simulink library "kukaslxctrl"  (R2016b)
settings: Solver=ode45  StartTime=0.0  StopTime=10.0  RelTol=1e-3  EnableMultiTasking=on
undefined symbols (not defined in the file): dcpctrl, getInitState, Standard_Devices, UDP_Protocol
libraries: simulink x2, sldrtlib x2
settings Model: Creator=julianleland  LastModifiedBy=dcp
settings DataIOCC: LimitDataPoints=on
settings OptimizationCC: LifeSpan=inf
settings DebuggingCC: AllowSymbolicDim=off  SFUnexpectedBacktrackingDiag=warning  SFNoUnconditionalDefaultTransitionDiag=warning  SFExecutionAtInitializationDiag=none
settings GRTTargetCC: TargetLangStandard=C89/C90 (ANSI)  GeneratePreprocessorConditionals=Disable all
settings ConfigComp: CovMetricSettings=dw  CovHtmlReporting=on  CovSaveCumulativeToWorkspaceVar=on  CovSaveSingleToWorkspaceVar=on  CovExternalEMLEnable=off

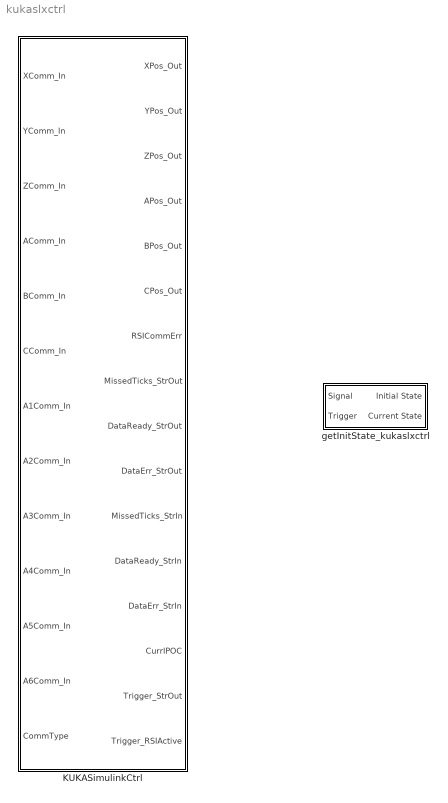
== system kukaslxctrl ==
  KUKASimulinkCtrl : Subsystem  mask(KUKASimulinkCtrl){}
      mask help:
      | This block produces an interface for communicating with KUKA robots using KRC4 and RSI. This block is currently in development, so not all inputs and outputs are usable yet!
      |
      | Notes:
      |  - This system assumes relative motion commands by default: e.g., a command of 1 sent to XComm_In will tell the KUKA to move at 1 mm/.004 sec (= 250 mm/sec - don't do this, too fast!!).
      |  - You will need to configure the Stream Input and Stream Output blocks inside this block - as well as the KUKA RSI files - to match your network configuration.
      |  - This block requires the Simulink Desktop Real-Time blockset to operate.
      |
      | Please see help for detailed information on inputs and outputs.
      mask Help:
      | INPUTS:
      |  - XComm_In, etc.: Task-space (XYZABC) commands to send to KUKA.
      |  - A1Comm_In, etc.: Joint-space commands to send to KUKA. NOT CURRENTLY FUNCTIONAL.
      |  - CommType: Flag to indicate whether using task-space or joint-space commands. NOT CURRENTLY FUNCTIONAL.
      | 
      | OUTPUTS:
      |  - XPos_Out, etc.: Task-space positions.
      |  - RSICommErr: Eventually will report if there's an error in creating an RSI packet - currently does nothing.
      |  - MissedTicks_StrOut: Missed ticks from UDP Stream Output block.
      |  - DataReady_StrOut: Data Ready flag from UDP Stream Output block.
      |  - DataErr_StrOut: Data Error flag from UDP Stream Output block.
      |  - MissedTicks_StrIn: Missed ticks from UDP Stream Input block.
      |  - DataReady_StrIn: Data Ready flag from UDP Stream Input block.
      |  - DataErr_StrIn: Data Error flag from UDP Stream Input block.
      |  - CurrIPOC: Reports the IPOC from the last received packet.
      |  - Trigger_StrOut: Trigger flag indicating when stream output has been turned on (after system has received first packet from KUKA).
      |  - Trigger_RSIActive: Trigger flag indicating when a numerical (non-NaN) IPOC value has been received.
      | 
      | DEPENDENCIES: Requires Simulink Desktop Real-Time.
      | 
      | NOTES: None.
  getInitState_kukaslxctrl : Subsystem  AncestorBlock=dcpctrl/getInitState  mask(Initial State Capture){}
      mask help:
      | Captures state of signal at time that trigger input is set high. Outputs captured state, as well as current signal. A common use of this block is to capture the initial state of a signal, and then subtract the initial state from the current state, giving a measure of how much a signal has changed over time.
      |
      | INPUTS:
      |  - Signal: Signal to capture state of.
      |  - Trigger: Signal carrying trigger to set state capture. Captures on rising edge. A step signal is a good choice for a trigger.
      |
      | OUTPUTS:
      |  - Initial State: State of signal at time when trigger rising edge is detected.
      |  - Current State: Signal (passed through).
      |
      | DEPENDENCIES: None
      |
      | NOTES: This is a convenience function included to support the example kukaslxctrl.slx

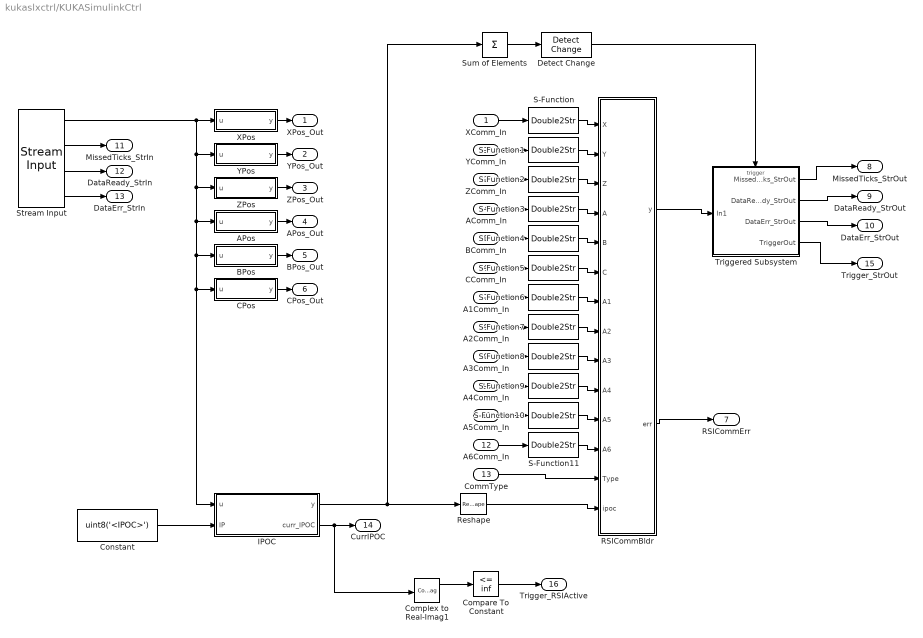
== system kukaslxctrl/KUKASimulinkCtrl ==
  XComm_In : Inport
  YComm_In : Inport  Port=2
  ZComm_In : Inport  Port=3
  AComm_In : Inport  Port=4
  BComm_In : Inport  Port=5
  CComm_In : Inport  Port=6
  A1Comm_In : Inport  Port=7
  A2Comm_In : Inport  Port=8
  A3Comm_In : Inport  Port=9
  A4Comm_In : Inport  Port=10
  A5Comm_In : Inport  Port=11
  A6Comm_In : Inport  Port=12
  CommType : Inport  Port=13
  APos : MATLAB Function  TreatAsAtomicUnit=on
  BPos : MATLAB Function  TreatAsAtomicUnit=on
  CPos : MATLAB Function  TreatAsAtomicUnit=on
  Compare To Constant : simulink/Logic and Bit Operations/Compare To Constant  relop=<=  const=inf  OutDataTypeStr=boolean
  Complex to Real-Imag1 : ComplexToRealImag
  Constant : Constant  Value=uint8('<IPOC>')
  Detect Change : simulink/Logic and Bit Operations/Detect Change  vinit=0  OutDataTypeStr=boolean
  IPOC : MATLAB Function  TreatAsAtomicUnit=on
  RSICommBldr : MATLAB Function  TreatAsAtomicUnit=on
  Reshape : Reshape
  S-Function{,1..11} (12 alike) : S-Function  FunctionName=Double2Str  SFunctionDeploymentMode=off  EnableBusSupport=off
  Stream Input : sldrtlib/Stream Input  SampleTime=-1  MaxMissedTicks=10  ShowMissedTicks=on  YieldWhenWaiting=on  DrvName=Standard_Devices/UDP_Protocol  DrvAddress=27277  DrvOptions=[174338149 53453]  DataTypes='238*uint16'  FormatString=repmat('%c',1,238)  Terminator='/Rob>'  ShowReady=on  ShowError=on
      settings: AttributesFormatString=Standard Devices\nUDP Protocol [6A8Dh]
  Sum of Elements : Sum  Inputs=+  CollapseMode=Specified dimension  CollapseDim=2
  Triggered Subsystem : Subsystem  TreatAsAtomicUnit=on
  XPos : MATLAB Function  TreatAsAtomicUnit=on
  YPos : MATLAB Function  TreatAsAtomicUnit=on
  ZPos : MATLAB Function  TreatAsAtomicUnit=on
  XPos_Out : Outport
  YPos_Out : Outport  Port=2
  ZPos_Out : Outport  Port=3
  APos_Out : Outport  Port=4
  BPos_Out : Outport  Port=5
  CPos_Out : Outport  Port=6
  RSICommErr : Outport  Port=7
  MissedTicks_StrOut : Outport  Port=8
  DataReady_StrOut : Outport  Port=9
  DataErr_StrOut : Outport  Port=10
  MissedTicks_StrIn : Outport  Port=11
  DataReady_StrIn : Outport  Port=12
  DataErr_StrIn : Outport  Port=13
  CurrIPOC : Outport  Port=14
  Trigger_StrOut : Outport  Port=15
  Trigger_RSIActive : Outport  Port=16
  wires:
  YComm_In/1 -> S-Function1/1
  BPos/1(y) -> BPos_Out/1
  CComm_In/1 -> S-Function5/1
  ZComm_In/1 -> S-Function2/1
  AComm_In/1 -> S-Function3/1
  BComm_In/1 -> S-Function4/1
  A6Comm_In/1 -> S-Function11/1
  RSICommBldr/2(err) -> RSICommErr/1
  A5Comm_In/1 -> S-Function10/1
  XPos/1(y) -> XPos_Out/1
  A2Comm_In/1 -> S-Function7/1
  A4Comm_In/1 -> S-Function9/1
  APos/1(y) -> APos_Out/1
  A3Comm_In/1 -> S-Function8/1
  YPos/1(y) -> YPos_Out/1
  A1Comm_In/1 -> S-Function6/1
  ZPos/1(y) -> ZPos_Out/1
  XComm_In/1 -> S-Function/1
  CPos/1(y) -> CPos_Out/1
  Stream Input/3 -> DataReady_StrIn/1
  S-Function/1 -> RSICommBldr/1(X)
  Stream Input/2 -> MissedTicks_StrIn/1
  Stream Input/1 -> IPOC/1(u), CPos/1(u), BPos/1(u), APos/1(u), ZPos/1(u), YPos/1(u), XPos/1(u)
  RSICommBldr/1(y) -> Triggered Subsystem/1(In1)
  IPOC/1(y) -> Sum of Elements/1, Reshape/1
  Constant/1 -> IPOC/2(IP)
  S-Function1/1 -> RSICommBldr/2(Y)
  S-Function2/1 -> RSICommBldr/3(Z)
  S-Function3/1 -> RSICommBldr/4(A)
  S-Function4/1 -> RSICommBldr/5(B)
  S-Function5/1 -> RSICommBldr/6(C)
  S-Function6/1 -> RSICommBldr/7(A1)
  S-Function7/1 -> RSICommBldr/8(A2)
  S-Function8/1 -> RSICommBldr/9(A3)
  S-Function9/1 -> RSICommBldr/10(A4)
  S-Function10/1 -> RSICommBldr/11(A5)
  S-Function11/1 -> RSICommBldr/12(A6)
  Triggered Subsystem/1(MissedTicks_StrOut) -> MissedTicks_StrOut/1
  Triggered Subsystem/2(DataReady_StrOut) -> DataReady_StrOut/1
  Triggered Subsystem/3(DataErr_StrOut) -> DataErr_StrOut/1
  Stream Input/4 -> DataErr_StrIn/1
  IPOC/2(curr_IPOC) -> Complex to Real-Imag1/1, CurrIPOC/1
  Reshape/1 -> RSICommBldr/14(ipoc)
  CommType/1 -> RSICommBldr/13(Type)
  Triggered Subsystem/4(TriggerOut) -> Trigger_StrOut/1
  Detect Change/1 -> Triggered Subsystem/Trigger
  Sum of Elements/1 -> Detect Change/1
  Compare To Constant/1 -> Trigger_RSIActive/1
  Complex to Real-Imag1/1 -> Compare To Constant/1

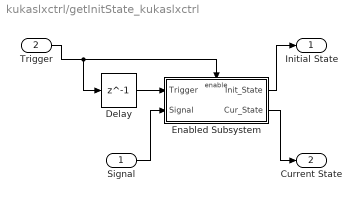
== system kukaslxctrl/getInitState_kukaslxctrl ==
  Signal : Inport
  Trigger : Inport  Port=2
  Delay : Delay  DelayLength=1  InitialCondition=0
  Enabled Subsystem : Subsystem  TreatAsAtomicUnit=on
  Initial State : Outport
  Current State : Outport  Port=2
  wires:
  Delay/1 -> Enabled Subsystem/1(Trigger)
  Trigger/1 -> Enabled Subsystem/Enable, Delay/1
  Enabled Subsystem/2(Cur_State) -> Current State/1
  Enabled Subsystem/1(Init_State) -> Initial State/1
  Signal/1 -> Enabled Subsystem/2(Signal)

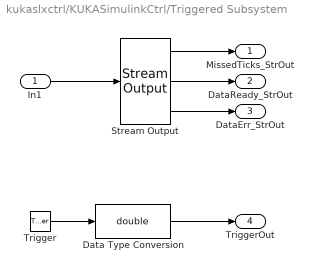
== system kukaslxctrl/KUKASimulinkCtrl/Triggered Subsystem ==
  In1 : Inport
  Trigger : TriggerPort  VariantControl=Variant  ShowOutputPort=on
  Data Type Conversion : DataTypeConversion  OutDataTypeStr=double
  Stream Output : sldrtlib/Stream Output  SampleTime=inf  MaxMissedTicks=10  ShowMissedTicks=on  YieldWhenWaiting=off  DrvName=Standard_Devices/UDP_Protocol  DrvAddress=27277  DrvOptions=[174338149 53453]  PortSizes=282  FormatString=repmat('%c',1,282)  ShowReady=on  ShowError=on  InitialValue=[]  FinalValue=[]
      settings: AttributesFormatString=Standard Devices\nUDP Protocol [6A8Dh]
  MissedTicks_StrOut : Outport
  DataReady_StrOut : Outport  Port=2
  DataErr_StrOut : Outport  Port=3
  TriggerOut : Outport  Port=4
  wires:
  Stream Output/1 -> MissedTicks_StrOut/1
  Stream Output/2 -> DataReady_StrOut/1
  Stream Output/3 -> DataErr_StrOut/1
  In1/1 -> Stream Output/1
  Data Type Conversion/1 -> TriggerOut/1
  Trigger/1 -> Data Type Conversion/1

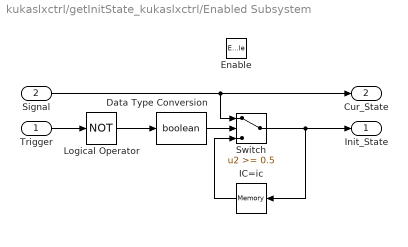
== system kukaslxctrl/getInitState_kukaslxctrl/Enabled Subsystem ==
  Trigger : Inport
  Signal : Inport  Port=2
  Enable : EnablePort  StatesWhenEnabling=reset
  Data Type Conversion : DataTypeConversion  OutDataTypeStr=boolean
  IC=ic : Memory  LinearizeAsDelay=on
  Logical Operator : Logic  Operator=NOT  AllPortsSameDT=off  OutDataTypeStr=boolean
  Switch : Switch  Threshold=0.5  SaturateOnIntegerOverflow=on  InputSameDT=on
  Init_State : Outport
  Cur_State : Outport  Port=2
  wires:
  Signal/1 -> Switch/1, Cur_State/1
  Logical Operator/1 -> Data Type Conversion/1
  IC=ic/1 -> Switch/3
  Switch/1 -> Init_State/1, IC=ic/1
  Data Type Conversion/1 -> Switch/2
  Trigger/1 -> Logical Operator/1

== matlab function kukaslxctrl/KUKASimulinkCtrl/XPos ==
  data: u input; y output
function y = fcn(u)
%#codegen

% Convert input into characters.
string = char(u);

% Locate start of X and Y strings
indx_X = strfind(string','X=');
indx_Y = strfind(string','Y=');

% Once X and Y strings have been located, grab the intervening characters
% (the X position). Otherwise, set to 0.
if ~isempty(indx_X)
    str_X = string((indx_X(1)+3):(indx_Y(1)-3));
    doub_X = str2double(str_X);
    y = doub_X;
else
    y = 0.0;
% TODO: Is this safe? Probably - if we're in abs mode and we command zero
% from some far distance away, it will cause a fault.
end

== matlab function kukaslxctrl/KUKASimulinkCtrl/RSICommBldr ==
  data: X input; Y input; Z input; A input; B input; C input; A1 input; A2 input; A3 input; A4 input; A5 input; A6 input; Type input; y output size=[1 282]; ipoc input; err output
function [y, err] = fcn(X,Y,Z,A,B,C,A1,A2,A3,A4,A5,A6,Type,ipoc)
%#codegen

err = 0; % Default: define no error state.

%{
% Check whether we're inputting a RKorr or AKorr
switch Type
    case 82 % Either 'R' or 'r' passed in as uint8 - 82 or 114
        s1 = uint8('<Sen Type="ImFree"><RKorr ');
        s2 = uint8('X="');
        s3 = uint8('" Y="');
        s4 = uint8('" Z="');
        s5 = uint8('" A="');
        s6 = uint8('" B="');
        s7 = uint8('" C="');
        s8 = uint8('" /><IPOC>');
        s9 = uint8('</IPOC></Sen>');
        y = [s1 s2 X' s3 Y' s4 Z' s5 A' s6 B' s7 C' s8 ipoc' s9]
    case 65 % Either 'A' or 'a' passed in as uint8 - 65 or 97
        y = uint8('<Sen Type="ImFree"><RKorr '); % DUMMY - write correct string for analog input here instead
    otherwise
        y = uint8(''); % Send empty string so that KUKA gets upset
        err = 1; % Set error flag to 1
%}

% Set up crlf string
crlf = [char(13) char(10)]; % Carriage return plus line feed

% Process IPOC to remove leading x's & add extra whitespace
coder.varsize('ipoc_char');
ipoc_char = char(ipoc');
ipoc_char_orig = ipoc_char;
ipoc_char([ipoc_char == 'x']) = [];
numremoved = length(ipoc_char_orig)-length(ipoc_char);
extChars = (ones(1,numremoved)*32)';
ipoc_uint = uint8(ipoc_char)';

% Create rest of string
s1 = uint8(['<Sen Type="ImFree">' crlf]);
s1p1 = uint8(['<EStr></EStr>' crlf]);
s1p2 = uint8(['<Tech T21="1.09" T22="2.08" T23="3.07" T24="4.06" T25="5.05" T26="6.04" T27="7.03" T28="8.02" T29="9.01" T210="10.00" />' crlf]);
s1p3 = uint8('<RKorr ');
s2 = uint8('X="');
s3 = uint8('" Y="');
s4 = uint8('" Z="');
s5 = uint8('" A="');
s6 = uint8('" B="');
s7 = uint8('" C="');
s8 = uint8(['" />' crlf]);
s9 = uint8(['<DiO>125</DiO>' crlf]);
s10 = uint8('<IPOC>');
s11 = uint8(['</IPOC>' crlf]);
s12 = uint8('</Sen>');
%{
s8 = uint8('" /><IPOC>');
s9 = uint8('</IPOC><DiO>125</DiO></Sen>');
%}
y_temp = [s1 s1p1 s1p2 s1p3 s2 X' s3 Y' s4 Z' s5 A' s6 B' s7 C' s8 s9 s10 ipoc_uint' s11 s12 extChars'];
y = uint8(y_temp(1:282));
end

== matlab function kukaslxctrl/KUKASimulinkCtrl/YPos ==
  data: u input; y output
function y = fcn(u)
%#codegen

% Convert input into characters.
string = char(u);

% Locate start of X and Y strings
indx_Y = strfind(string','Y=');
indx_Z = strfind(string','Z=');

% Once X and Y strings have been located, grab the intervening characters
% (the X position). Otherwise, set to 0.
if ~isempty(indx_Y)
    str_Y = string((indx_Y(1)+3):(indx_Z(1)-3));
    doub_Y = str2double(str_Y);
    y = doub_Y;
else
    y = 0.0;
% TODO: Is this safe? Probably - if we're in abs mode and we command zero
% from some far distance away, it will cause a fault.
end

== matlab function kukaslxctrl/KUKASimulinkCtrl/ZPos ==
  data: u input; y output
function y = fcn(u)
%#codegen

% Convert input into characters.
string = char(u);

% Locate start of X and Y strings
indx_Z = strfind(string','Z=');
indx_A = strfind(string','A=');

% Once X and Y strings have been located, grab the intervening characters
% (the X position). Otherwise, set to 0.
if ~isempty(indx_Z)
    str_Z = string((indx_Z(1)+3):(indx_A(1)-3));
    doub_Z = str2double(str_Z);
    y = doub_Z;
else
    y = 0.0;
% TODO: Is this safe? Probably - if we're in abs mode and we command zero
% from some far distance away, it will cause a fault.
end

== matlab function kukaslxctrl/KUKASimulinkCtrl/APos ==
  data: u input; y output
function y = fcn(u)
%#codegen

% Convert input into characters.
string = char(u);

% Locate start of X and Y strings
indx_A = strfind(string','A=');
indx_B = strfind(string','B=');

% Once X and Y strings have been located, grab the intervening characters
% (the X position). Otherwise, set to 0.
if ~isempty(indx_A)
    str_A = string((indx_A(1)+3):(indx_B(1)-3));
    doub_A = str2double(str_A);
    y = doub_A;
else
    y = 0.0;
% TODO: Is this safe? Probably - if we're in abs mode and we command zero
% from some far distance away, it will cause a fault.
end

== matlab function kukaslxctrl/KUKASimulinkCtrl/BPos ==
  data: u input; y output
function y = fcn(u)
%#codegen

% Convert input into characters.
string = char(u);

% Locate start of X and Y strings
indx_B = strfind(string','B=');
indx_C = strfind(string','C=');

% Once X and Y strings have been located, grab the intervening characters
% (the X position). Otherwise, set to 0.
if ~isempty(indx_B)
    str_B = string((indx_B(1)+3):(indx_C(1)-3));
    doub_B = str2double(str_B);
    y = doub_B;
else
    y = 0.0;
% TODO: Is this safe? Probably - if we're in abs mode and we command zero
% from some far distance away, it will cause a fault.
end

== matlab function kukaslxctrl/KUKASimulinkCtrl/CPos ==
  data: u input; y output
function y = fcn(u)
%#codegen

% Convert input into characters.
string = char(u);

% Locate start of X and Y strings
indx_C = strfind(string','C=');
indx_RSol = strfind(string','/><AIPos');

% Once X and Y strings have been located, grab the intervening characters
% (the X position). Otherwise, set to 0.
if ~isempty(indx_C)
    str_C = string((indx_C(1)+3):(indx_RSol(1)-3));
    doub_C = str2double(str_C);
    y = doub_C;
else
    y = 0.0;
% TODO: Is this safe? Probably - if we're in abs mode and we command zero
% from some far distance away, it will cause a fault.
end

== matlab function kukaslxctrl/KUKASimulinkCtrl/IPOC ==
  data: u input; y output; IP input; curr_IPOC output
function [y, curr_IPOC] = fcn(u, IP)
%#codegen

pos = 1;
pos_end = 2;
startStrLen = 6; % Length of IPOC start string. Hard-coded for speed
lenU = length(u);
%disp(['Reading input:' u']);

for i = 1:length(u)-startStrLen
    % Compare every set of 6 elements to IPOC start string. If their sum is
    % 6, we've found the start of the string.
    if (sum(u(i:i+(startStrLen-1)) == IP) == 6)
        pos = i+startStrLen;
    end
end

for i = pos:lenU
    if (u(i) == 60) % Search for next '<' character after IPOC
        pos_end = i-1;
        break; % Need to stop searching after we've found the end of the string
    end
end

% Pad IPOC with x's

ipocval = u(pos:pos_end);
ipoclen = length(ipocval);

ipoctemp = ones(1,10)*120; % Pad beginning of string with x's to show that this is a null character.
for n = 10:-1:10-length(ipocval)+1
    ipoctemp(n) = ipocval(end-(10-n));
end

curr_IPOC = str2double(char(ipocval));
y = uint8(ipoctemp(1:10));
